simulink model "EEPROM_SmartWheels"  (R2024b)
settings: Solver=FixedStepDiscrete  StartTime=0.0  StopTime=10.0  RelTol=1e-3
InitFcn:
  | mbd_s32k_consistency_checks(bdroot(gcs));
undefined symbols (not defined in the file): LQFP
libraries: mbd_s32k1xx_ec_toolbox x6
settings Model: Creator=Shreyas  LastModifiedBy=Shreyas
settings DataIOCC: ExternalInput=off  InitialState=off  SaveOutput=off  SignalLogging=off  SaveTime=off
settings OptimizationCC: DefaultParameterBehavior=Inlined  EnhancedBackFolding=on  PassReuseOutputArgsAs=Individual arguments  ZeroExternalMemoryAtStartup=off  ZeroInternalMemoryAtStartup=off  OptimizeBlockOrder=speed  DifferentSizesBufferReuse=on  OptimizationCustomize=off  EfficientTunableParamExpr=on
settings DebuggingCC: InheritedTsInSrcMsg=none  SingleTaskRateTransMsg=error  ParameterTunabilityLossMsg=error  UnconnectedInputMsg=error  UnconnectedOutputMsg=error  UnconnectedLineMsg=error  UnknownTsInhSupMsg=error
settings HardwareCC: ProdBitPerPointer=32  ProdBitPerSizeT=32  ProdBitPerPtrDiffT=32  ProdLargestAtomicInteger=Long  ProdLargestAtomicFloat=Double  ProdWordSize=32  ProdHWDeviceType=ARM Compatible->ARM Cortex
settings SFSimCC: MATLABDynamicMemAlloc=off
settings RTWCC: Description=Model Based Design Toolbox S32K1xx Code Generation Target  SystemTargetFile=mbd_s32k.tlc  MakeCommand=mbd_s32k_make_rtw COPY_MDLREF_INCLUDES=0  TemplateMakefile=mbd_s32k.tmf  PostCodeGenCommand=fix_mbd_makefiles
settings CodeAppCC: ForceParamTrailComments=on  IgnoreCustomStorageClasses=off  OperatorAnnotations=on  SimulinkDataObjDesc=on  SFDataObjDesc=on  InsertBlockDesc=on
settings STFCustomTargetCC: TargetLangStandard=C99 (ISO)  MultiwordLength=256  CombineOutputUpdateFcns=on  ERTCustomFileBanners=on  SupportContinuousTime=off  SupportNonInlinedSFcns=off  RemoveResetFunc=on  MATLABClassNameForMDSCustomization=Simulink.SoftwareTarget.ERTCustomization  SystemTargetFile=mbd_s32k.tlc
settings ERTTargetCC: TargetLangStandard=C99 (ISO)  ParMdlRefBuildCompliant=off  CompOptLevelCompliant=off  ConcurrentExecutionCompliant=off  ModelStepFunctionPrototypeControlCompliant=off  CPPClassGenCompliant=off  UseToolchainInfoCompliant=off  ERTSrcFileBannerTemplate=mbd_ert_code_template.cgt  ERTHdrFileBannerTemplate=mbd_ert_code_template.cgt  ERTDataSrcFileTemplate=mbd_ert_code_template.cgt  ERTDataHdrFileTemplate=mbd_ert_code_template.cgt  ERTCustomFileTemplate=example_file_process.tlc

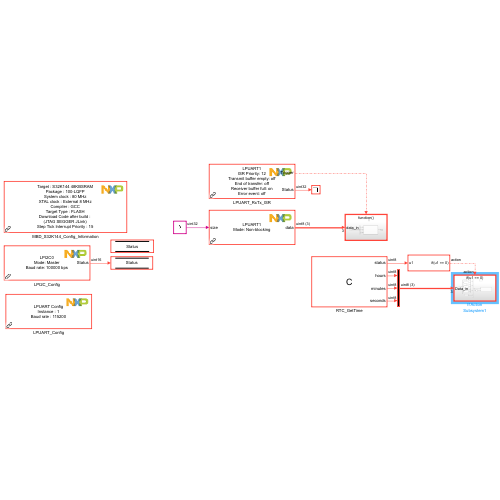
[thumbnail: Simulink's stored preview of the top-level diagram]
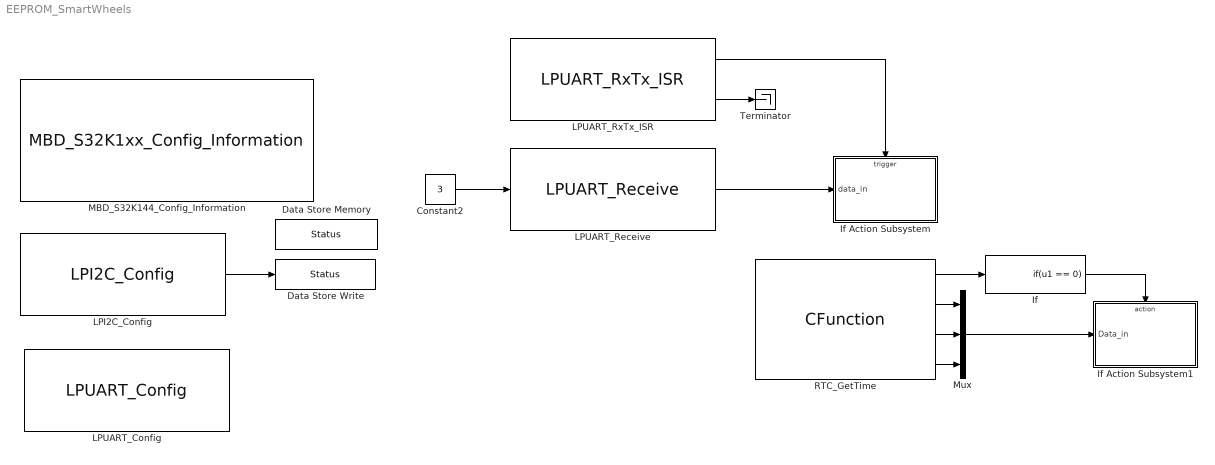
== system EEPROM_SmartWheels ==
  Constant2 : Constant  Value=3  OutDataTypeStr=uint32
  Data Store Memory : DataStoreMemory  DataStoreName=Status  WriteAfterWriteMsg=warning  ShowAdditionalParam=off
  Data Store Write : DataStoreWrite  DataStoreName=Status  IndexOptions=Index vector (dialog)  Indices=1  OutputSizes=1
  If : If  IfExpression=u1 == 0  ShowElse=off
  If Action Subsystem : Subsystem  TreatAsAtomicUnit=on
  If Action Subsystem1 : Subsystem  TreatAsAtomicUnit=on
  LPI2C_Config : mbd_s32k1xx_ec_toolbox/Communication Blocks/I2C Blocks/LPI2C_Config  instance=0  mode=Master  opmode=Standard (up to 100 kbit/s)  bdr=100000  addr=1  is10bitaddr=off  status=on  sda=PTA2: [LPI2C0_SDA | LPI2C Data I/O]  scl=PTA3: [LPI2C0_SCL | LPI2C Clock I/O]
  LPUART_Config : mbd_s32k1xx_ec_toolbox/Communication Blocks/UART Blocks/LPUART_Config  Priority=1  instance=1  baudrate=115200  custom_baudrate=1000000  databits=8  parity=None  sbns=1  bothedge=rising edge  rxinv=off  txinv=off  show_adv_opts=on  brk13=10 - 13 bit times  lbkde=10 - 13 bit times  rx=PTC6: [LPUART1_RX | Receive]  tx=PTC7: [LPUART1_TX | Transmit]
  LPUART_Receive : mbd_s32k1xx_ec_toolbox/Communication Blocks/UART Blocks/LPUART_Receive  instance=1  receive_mode=Non-blocking  timeout=500
  LPUART_RxTx_ISR : mbd_s32k1xx_ec_toolbox/Communication Blocks/UART Blocks/LPUART_RxTx_ISR  instance=1  prio=12  tie=off  tcie=off  rie=on  ilie=off
  MBD_S32K144_Config_Information : mbd_s32k1xx_ec_toolbox/MBD_S32K1xx_Config_Information  mbdt_ver=0  disp_str=|  config_params=[]  mcu_target_name=S32K144  mcu_target_package=100-LQFP  mcu_target_sram_size=48KB  mcu_system_clock_freq=80  mcu_xtal_freq=External 8  mcu_steptick_timer=LPIT Channel 0  mcu_steptick_prio=15  ds_import_enable=on  target_compiler=GCC  target_memory=FLASH  gcc_target_compile_opts=-mthumb -mfloat-abi=hard -mfpu=fpv4-sp-d16 -O1 -g -gstrict-dwarf  gcc_target_assemble_opts=-mthumb -mfloat-abi=hard -mfpu=fpv4-sp-d16 -g  gcc_target_link_opts=-mthumb -mfloat-abi=hard -mfpu=fpv4-sp-d16  gcc_target_default_lcf=on  gcc_target_user_lcf=S32K144_48_flash.ld  ghs_target_compile_opts=-cpu=cortexm4f -thumb -fpu=vfpv4_d16 -fsingle -Ogeneral -Wundef -Wimplicit-int -Wshadow -Wtrigraphs --no_commons --gnu_asm -gnu99 -gdwarf-2 -G  ghs_target_assemble_opts=-cpu=cortexm4f -fpu=vfpv4_d16  ghs_target_link_opts=-cpu=cortexm4f -thumb -fpu=vfpv4_d16  ghs_target_default_lcf=on  ghs_target_user_lcf=S32K144_48_flash.ld  iar_target_compile_opts=--cpu=Cortex-M4F --thumb --fpu=VFPv4_sp -Ol -e --debug --dlib_config normal  iar_target_assemble_opts=--cpu Cortex-M4F --thumb --fpu VFPv4_sp  iar_target_link_opts=--no_exceptions --vfe --inline  iar_target_default_lcf=on  iar_target_user_lcf=S32K144_48_flash.icf  pil_download_enable=off  rbl_download_enable=on  rbl_start_delay=5000  rbl_download_interface=JTAG  rbl_restart_request=off  rbl_com_port=Custom  rbl_com_port_custom=COM1  pil_download_rate=115200  pil_download_rate_custom=115200  pil_opensda_drive=Custom  pil_opensda_drive_custom=D  jtag_interface=SEGGER JLink  jlink_default_path=on  jlink_user_path=C:\Program Files\SEGGER\JLink\  pil_uart_instance=1  pil_uart_rx=PTC6: [LPUART1_RX | Receive]  pil_uart_tx=PTC7: [LPUART1_TX | Transmit]  FTM_PWM_PcrCheckEnDis=on  FTM_Input_Edge_Inputs_PcrCheckEnDis=on  FTM_Dual_Edge_Inputs_PcrCheckEnDis=on  FTM_Quadrature_Inputs_PcrCheckEnDis=on  FTM_Hall_Sensor_Inputs_PcrCheckEnDis=on  LPTMR_PcrCheckEnDis=on  PIT_PcrCheckEnDis=on  RTC_PcrCheckEnDis=on  FlexCAN_PcrCheckEnDis=on  LIN_PcrCheckEnDis=on  FlexIO_PcrCheckEnDis=on  LPI2C_PcrCheckEnDis=on  LPSPI_PcrCheckEnDis=on  LPUART_PcrCheckEnDis=on  CMP_PcrCheckEnDis=on  GPIO_OutputPcrCheckEnDis=on  GPIO_InputPcrCheckEnDis=on  SBC_PcrCheckEnDis=on  BMS_PcrCheckEnDis=on  AMMCLIB_PcrCheckEnDis=on  FM_PcrCheckEnDis=on  Profile_PcrCheckEnDis=on  ConfigParams_PcrCheckEnDis=on  ModelRef_PcrCheckEnDis=on  PDB0_PcrCheckEnDis=on  CSEc_PcrCheckEnDis=on  eDMA_PcrCheckEnDis=on  FLASH_PcrCheckEnDis=on  ADC_PcrCheckEnDis=on  WDOG_PcrCheckEnDis=on
      | Target : S32K144-64KB_SRAM
      | Package : 100-pin
      | System clock : 80 MHz
      | XTAL clock : External 8 MHz
      | Compiler : IAR
      | Target Type : FLASH
      | Download Code after build : off
      | Step Tick Interrupt Priority : 15
  Mux : Mux  Inputs=3
  RTC_GetTime : CFunction  OutputCode=|  CodegenOutputCode=|  SimCustomHeaderFile=ds3231.h  SimCustomSourceFile=ds3231.c  CustomHeaderFile=ds3231.h  CustomSourceFile=ds3231.c  CustomCodeIsMultiInstantiable=on
      OutputCode=|
      | /* Read Time: Hours (0-23), Minutes (0-59), Seconds (0-59) */
      | status = DS3231_GetTimeScalars(&hours, &minutes, &seconds);
      CodegenOutputCode=|
      | /* Read Time: Hours (0-23), Minutes (0-59), Seconds (0-59) */
      | status = DS3231_GetTimeScalars(&hours, &minutes, &seconds);
  Terminator : Terminator
  wires:
  LPI2C_Config/1 -> Data Store Write/1
  RTC_GetTime/1 -> If/1
  If/1 -> If Action Subsystem1/Action
  Mux/1 -> If Action Subsystem1/1(Data_in)
  LPUART_RxTx_ISR/1 -> If Action Subsystem/Trigger
  LPUART_Receive/1 -> If Action Subsystem/1(data_in)
  Constant2/1 -> LPUART_Receive/1
  LPUART_RxTx_ISR/2 -> Terminator/1
  RTC_GetTime/2 -> Mux/1
  RTC_GetTime/3 -> Mux/2
  RTC_GetTime/4 -> Mux/3

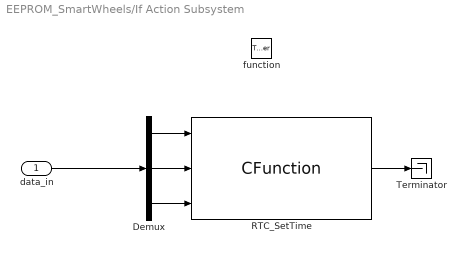
== system EEPROM_SmartWheels/If Action Subsystem ==
  data_in : Inport
  function : TriggerPort  TriggerType=function-call  VariantControl=(inherit)
  Demux : Demux  Outputs=3
  RTC_SetTime : CFunction  OutputCode=|  CodegenOutputCode=|  SimCustomHeaderFile=ds3231.h  SimCustomSourceFile=ds3231.c  CustomHeaderFile=ds3231.h  CustomSourceFile=ds3231.c  CustomCodeIsMultiInstantiable=on
      OutputCode=|
      | /* Write Time to DS3231 */
      | status = DS3231_SetTimeScalars(hours, minutes, seconds);
      CodegenOutputCode=|
      | /* Write Time to DS3231 */
      | status = DS3231_SetTimeScalars(hours, minutes, seconds);
  Terminator : Terminator
  wires:
  RTC_SetTime/1 -> Terminator/1
  Demux/2 -> RTC_SetTime/2
  Demux/1 -> RTC_SetTime/1
  Demux/3 -> RTC_SetTime/3
  data_in/1 -> Demux/1

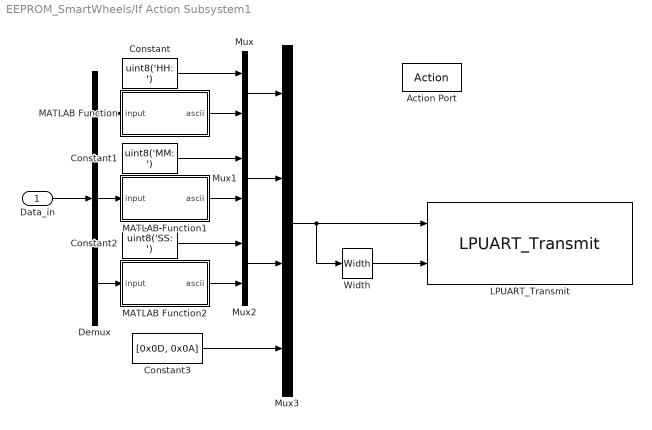
== system EEPROM_SmartWheels/If Action Subsystem1 ==
  Data_in : Inport
  Action Port : ActionPort  ActionPortLabel=if(u1 == 0)
  Constant : Constant  Value=uint8('HH: ')
  Constant1 : Constant  Value=uint8('MM: ')
  Constant2 : Constant  Value=uint8('SS: ')
  Constant3 : Constant  Value=[0x0D, 0x0A]
  Demux : Demux  Outputs=3
  LPUART_Transmit : mbd_s32k1xx_ec_toolbox/Communication Blocks/UART Blocks/LPUART_Transmit  instance=1  transmit_mode=Non-blocking  timeout=500  number=on
  MATLAB Function : MATLAB Function  TreatAsAtomicUnit=on
  MATLAB Function1 : MATLAB Function  TreatAsAtomicUnit=on
  MATLAB Function2 : MATLAB Function  TreatAsAtomicUnit=on
  Mux : Mux  Inputs=2
  Mux1 : Mux  Inputs=2
  Mux2 : Mux  Inputs=2
  Mux3 : Mux
  Width : Width  DataType=uint32
  wires:
  Width/1 -> LPUART_Transmit/2
  Data_in/1 -> Demux/1
  Demux/1 -> MATLAB Function/1(input)
  Constant/1 -> Mux/1
  Demux/2 -> MATLAB Function1/1(input)
  Constant1/1 -> Mux1/1
  Demux/3 -> MATLAB Function2/1(input)
  Constant2/1 -> Mux2/1
  MATLAB Function/1(ascii) -> Mux/2
  MATLAB Function1/1(ascii) -> Mux1/2
  MATLAB Function2/1(ascii) -> Mux2/2
  Constant3/1 -> Mux3/4
  Mux/1 -> Mux3/1
  Mux1/1 -> Mux3/2
  Mux2/1 -> Mux3/3
  Mux3/1 -> Width/1, LPUART_Transmit/1

== matlab function EEPROM_SmartWheels/If Action Subsystem1/MATLAB Function ==
  data: input input; ascii output
function ascii = decimalToASCII(input)
%#codegen
% Input : uint8
% Output: 1x3 uint8 ASCII array

ascii = uint8(zeros(1,3));

if input >= 100
    ascii(1) = uint8(floor(double(input) / 100) + 48);
    ascii(2) = uint8(mod(floor(double(input) / 10), 10) + 48);
    ascii(3) = uint8(mod(double(input), 10) + 48);

elseif input >= 10
    ascii(1) = uint8(floor(double(input) / 10) + 48);
    ascii(2) = uint8(mod(double(input), 10) + 48);

else
    ascii(1) = uint8(input + 48);
end

== matlab function EEPROM_SmartWheels/If Action Subsystem1/MATLAB Function2 ==
  data: input input; ascii output
function ascii = decimalToASCII(input)
%#codegen
% Input : uint8
% Output: 1x3 uint8 ASCII array

ascii = uint8(zeros(1,3));

if input >= 100
    ascii(1) = uint8(floor(double(input) / 100) + 48);
    ascii(2) = uint8(mod(floor(double(input) / 10), 10) + 48);
    ascii(3) = uint8(mod(double(input), 10) + 48);

elseif input >= 10
    ascii(1) = uint8(floor(double(input) / 10) + 48);
    ascii(2) = uint8(mod(double(input), 10) + 48);

else
    ascii(1) = uint8(input + 48);
end

== matlab function EEPROM_SmartWheels/If Action Subsystem1/MATLAB Function1 ==
  data: input input; ascii output
function ascii = decimalToASCII(input)
%#codegen
% Input : uint8
% Output: 1x3 uint8 ASCII array

ascii = uint8(zeros(1,3));

if input >= 100
    ascii(1) = uint8(floor(double(input) / 100) + 48);
    ascii(2) = uint8(mod(floor(double(input) / 10), 10) + 48);
    ascii(3) = uint8(mod(double(input), 10) + 48);

elseif input >= 10
    ascii(1) = uint8(floor(double(input) / 10) + 48);
    ascii(2) = uint8(mod(double(input), 10) + 48);

else
    ascii(1) = uint8(input + 48);
end
